simulink model "VFlexP_small"  (R2026a)
settings: Solver=ode23tb  StopTime=2  FixedStep=5e-5
model workspace (MAT data in the model file):
  DCop_DCBUCK : object (value not decoded)
  Grid_CCVSC_idx = [2; 3; 4; 5; 6; 7; 8; 9; 10; 11; 12]
  Grid_CCVSCs = 1
  Grid_CCVSCs_buses = 1
  Grid_CCVSCs_toM = [0 1 0 0 0 0 0 0 0 0 0 0 ... (781 elements, 71x11)]
  Grid_C_Lines = 0
  Grid_Cbuses = [0.00666666666667 0.00666666666667]
  Grid_DC : object (value not decoded)
  Grid_DCop_DCBUCK : object (value not decoded)
  Grid_DCop_DC_PES : object (value not decoded)
  Grid_DFIGs = 1
  Grid_DFIGs_buses = 1
  Grid_DGs : string (value not decoded)
  Grid_From_buses = 1
  Grid_GFls = 1
  Grid_GFls_buses = 1
  Grid_GFr_idx = 1
  Grid_GFrs = 1
  Grid_GFrs_buses = 1
  Grid_GFrs_toM = [1; 0]
  Grid_IG_idx = 1
  Grid_IGs = 1
  Grid_IGs_buses = 1
  Grid_IGs_toM = [1; 0; 0]
  Grid_L_Lines = 0.05
  Grid_L_Loads = [0 0]
  Grid_Lines_fromM : object (value not decoded)
  Grid_Lines_toM : object (value not decoded)
  Grid_Load_buses = [1; 2]
  Grid_Load_busesDC = []
  Grid_MSGs = 1
  Grid_MSGs_buses = 1
  Grid_Nbuses = 2
  Grid_PQ_gen = 3
  Grid_Ploads = [0.0075 0.0075]
  Grid_PloadsDC = []
  Grid_Ps_lf = 0.51232912
  Grid_Qloads = [0 0]
  Grid_Qs_lf = -0.00723209333333
  Grid_R_Lines = 0.005
  Grid_R_Loads = [2 2]
  Grid_R_Loads_DC = 0
  Grid_Rcf = [150 150]
  Grid_SCs = 1
  Grid_SCs_buses = 1
  Grid_SG_idx = 1
  Grid_SGs = 1
  Grid_SGs_buses = 1
  Grid_SGs_toM = [1; 0]
  Grid_To_buses = 2
  Grid_VCVSC_idx = [1; 2; 3; 4; 5; 6; 7; 8; 9; 10; 11; 12]
  Grid_VCVSCs = 1
  Grid_VCVSCs_buses = [1; 2; 3; 6; 8; 9; 12; 58; 59; 60; 63; 65]
  Grid_VCVSCs_toM = [1 0 0 0 0 0 0 0 0 0 0 0 ... (852 elements, 71x12)]
  Grid_VSM_idx = 2
  Grid_VSMs = 1
  Grid_VSMs_buses = 1
  Grid_VSMs_toM = [0; 1]
  Grid_admitt_matrix = [2.15353135314-19.7953135314i  -1.9801980198+19.801980198i; -1.9801980198+19.801980198i  2.15353135314-19.7953135314i]
  Grid_admitt_matrix_noloads = [1.98686468647-19.7953135314i  -1.9801980198+19.801980198i; -1.9801980198+19.801980198i  1.98686468647-19.7953135314i]
  Grid_bus = [1; 2]
  Grid_busDC_complexity = 1
  Grid_busDC_complexity_PF = 2
  Grid_bus_complexity = [1 1]
  Grid_bus_complexity_PF = [1 1]
  Grid_buses_lf = 1
  Grid_conductance_matrix = 0.00666666666667
  Grid_conductance_matrix_noloads = 0.00666666666667
  Grid_fref : object (value not decoded)
  Grid_gen_static_params : mBase (value not decoded)
  Grid_iPs_lf = 1.95187031336
  Grid_iQs_lf = -138.272551792
  Grid_iadmitt_matrix = [2.88165849328-0.0982918688642i  2.87905051706-0.123273862303i; 2.87905051706-0.123273862303i  2.88165849328-0.0982918688642i]
  Grid_iadmitt_matrix_noloads = [37.5012524798-37.4874983544i  37.4987475202-37.5125016456i; 37.4987475202-37.5125016456i  37.5012524798-37.4874983544i]
  Grid_iconductance_matrix = 150
  Grid_iconductance_matrix_noloads = 150
  Grid_init_OK_bool = 1
  Grid_intconv_PF : object (value not decoded)
  Grid_lf_op : op_report (value not decoded)
  Grid_lineDC_complexity = []
  Grid_lineDC_complexity_PF = []
  Grid_line_complexity = 1
  Grid_line_complexity_PF = 3
  Grid_loadDC_complexity = []
  Grid_loadDC_complexity_PF = []
  Grid_load_complexity = [3 3]
  Grid_load_complexity_PF = [4 4]
  Grid_opDC_CCVSC : object (value not decoded)
  Grid_opDC_VSM : object (value not decoded)
  Grid_opGFr : object (value not decoded)
  Grid_opVCVSC : object (value not decoded)
  Grid_op_CCVSC : object (value not decoded)
  Grid_op_IG : object (value not decoded)
  Grid_op_SG : object (value not decoded)
  Grid_op_VSM : object (value not decoded)
  Grid_shift_lines = 0
  Grid_tap_lines = 1
  Grid_v_buses_mod = [1 1]
  LinsysParamChangeStruct : Param1 (value not decoded)
  Lline = 0.01
  Rline = 1e-05
  linsys : object (value not decoded)
values from neighbouring files (symbols this model uses):
  block_idx = evalin(mdlWks, [bvarname Generators{i} '_idx'])    [fun_init_units_callback.m]
  Fb = areas    [fun_MATPOWER_to_Excel.m]
  Fi = evalin('base', get_param(block, 'Fi'))    [fun_init_GFr.m]    (also in fun_init_intconv_DC_VSM.m)
  Lf = evalin('base', get_param(block, 'Lf'))    [fun_init_GFr.m]    (also in fun_init_intconv_DC_VSM.m)
  Rf = evalin('base', get_param(block, 'Rf'))    [fun_init_GFr.m]    (also in fun_init_intconv_DC_VSM.m)
symbols that are objects in the model workspace (value not decoded): Grid_DCop_DC_PES, Grid_DCop_DCBUCK, Grid_op_CCVSC, Grid_op_IG, Grid_op_SG, Grid_op_VSM, Grid_opDC_CCVSC, Grid_opDC_VSM, Grid_opGFr, Grid_opVCVSC
undefined symbols (not defined in the file or in its folder): block_buses_DC, CCVSC_idx, Cf, costs, costs2, DFIGs_nodes, DiscIntNeverNeededParam, entity, From_nodes, grid_linsys, Grid_op_DFIG, Grid_op_DFIG_PQ, Grid_op_MSG, Grid_op_SC, Grid_op_VCVSC, Hv, initial_states_grid, Kic, Kiv, Kp_theta, Kp_w, Kpc, Kpv, last_send, Lc, m, Matrix_flux_to_i, mD, mp, MSGs_buses, Nbuses_DC, nq, op_VCVSC, Psche, Rc, rkq1, rkq2, SCs_buses, SCs_nodes, sec_control_structure, set_asked, set_DG_up, set_extra_satur, set_sending_cost, SGs_buses, SGs_nodes, Tf, To_nodes, VI_L, VI_R, WOF_Tf, xkq1, xkq2
libraries: simulink x1045, eeGeneralControl x12, eeTransforms x1, sl_discontinuities x1
(part 34 of 50)

== system VFlexP_small/Grid/Dynamic/Tertiary Control/MAS messages/ID6/Simulink Function14 ==
  set_cost_info : TriggerPort  TriggerType=function-call  IsSimulinkFunction=on  FunctionName=set_cost_info  FunctionVisibility=scoped  VariantControl=(inherit)
  cost : ArgIn  ArgumentName=cost
  Output : Outport
  wires:
  cost/1 -> Output/1

== system VFlexP_small/Grid/Dynamic/Tertiary Control/MAS messages/ID6/Simulink Function15 ==
  set_DG_up : TriggerPort  TriggerType=function-call  IsSimulinkFunction=on  FunctionName=set_DG_up  FunctionVisibility=scoped  VariantControl=(inherit)
  u : ArgIn  DisableCoverage=on  ArgumentName=u
  Output : Outport
  wires:
  u/1 -> Output/1

== system VFlexP_small/Grid/Dynamic/Tertiary Control/MAS messages/ID6/Simulink Function16 ==
  Input1 : Inport
  get_DG_up : TriggerPort  TriggerType=function-call  IsSimulinkFunction=on  FunctionName=get_DG_up  FunctionVisibility=scoped  VariantControl=(inherit)
  value : ArgOut  OutDataTypeStr=boolean  ArgumentName=value
  wires:
  Input1/1 -> value/1

== system VFlexP_small/Grid/Dynamic/Tertiary Control/MAS messages/ID6/Simulink Function17 ==
  set_neigh_ID : TriggerPort  TriggerType=function-call  IsSimulinkFunction=on  FunctionName=set_neigh_ID  FunctionVisibility=scoped  VariantControl=(inherit)
  u : ArgIn  DisableCoverage=on  ArgumentName=u
  Output : Outport
  wires:
  u/1 -> Output/1

== system VFlexP_small/Grid/Dynamic/Tertiary Control/MAS messages/ID6/Simulink Function18 ==
  Input1 : Inport
  get_neigh_ID : TriggerPort  TriggerType=function-call  IsSimulinkFunction=on  FunctionName=get_neigh_ID  FunctionVisibility=scoped  VariantControl=(inherit)
  value : ArgOut  ArgumentName=value
  wires:
  Input1/1 -> value/1

== system VFlexP_small/Grid/Dynamic/Tertiary Control/MAS messages/ID6/Simulink Function19 ==
  set_neigh_Opt : TriggerPort  TriggerType=function-call  IsSimulinkFunction=on  FunctionName=set_neigh_Opt  FunctionVisibility=scoped  VariantControl=(inherit)
  u : ArgIn  DisableCoverage=on  ArgumentName=u
  Output : Outport
  wires:
  u/1 -> Output/1

== system VFlexP_small/Grid/Dynamic/Tertiary Control/MAS messages/ID6/Simulink Function2 ==
  unpackage : TriggerPort  TriggerType=function-call  IsSimulinkFunction=on  FunctionName=unpackage  FunctionVisibility=scoped  VariantControl=(inherit)
  IC1 : InitialCondition
  IC2 : InitialCondition
  IC3 : InitialCondition  Value=v_buses_mod(buses_lf(IDnumber))
  IC4 : InitialCondition
  mpP~ : ArgIn  ArgumentName=P_s
  nqQ~ : ArgIn  Port=2  ArgumentName=Q_s
  v : ArgIn  Port=3  ArgumentName=v
  omega : ArgIn  Port=4  ArgumentName=omega
  Output2 : Outport
  Output3 : Outport  Port=2
  Output4 : Outport  Port=3
  Output5 : Outport  Port=4
  wires:
  omega/1 -> IC4/1  "omega"
  v/1 -> IC3/1  "v"
  nqQ~/1 -> IC2/1  "Q_s"
  mpP~/1 -> IC1/1  "P_s"
  IC1/1 -> Output2/1
  IC2/1 -> Output3/1
  IC4/1 -> Output5/1
  IC3/1 -> Output4/1

== system VFlexP_small/Grid/Dynamic/Tertiary Control/MAS messages/ID6/Simulink Function20 ==
  Input1 : Inport
  get_neigh_Opt : TriggerPort  TriggerType=function-call  IsSimulinkFunction=on  FunctionName=get_neigh_Opt  FunctionVisibility=scoped  VariantControl=(inherit)
  value : ArgOut  ArgumentName=value
  wires:
  Input1/1 -> value/1

== system VFlexP_small/Grid/Dynamic/Tertiary Control/MAS messages/ID6/Simulink Function21 ==
  set_sum_neigh_left : TriggerPort  TriggerType=function-call  IsSimulinkFunction=on  FunctionName=set_sum_neigh_left  FunctionVisibility=scoped  VariantControl=(inherit)
  u : ArgIn  DisableCoverage=on  ArgumentName=u
  Output : Outport
  wires:
  u/1 -> Output/1

== system VFlexP_small/Grid/Dynamic/Tertiary Control/MAS messages/ID6/Simulink Function22 ==
  set_Opt : TriggerPort  TriggerType=function-call  IsSimulinkFunction=on  FunctionName=set_Opt  FunctionVisibility=scoped  VariantControl=(inherit)
  u : ArgIn  DisableCoverage=on  ArgumentName=u
  Output : Outport
  wires:
  u/1 -> Output/1

== system VFlexP_small/Grid/Dynamic/Tertiary Control/MAS messages/ID6/Simulink Function23 ==
  Input1 : Inport
  get_sum_neigh_left : TriggerPort  TriggerType=function-call  IsSimulinkFunction=on  FunctionName=get_sum_neigh_left  FunctionVisibility=scoped  VariantControl=(inherit)
  value : ArgOut  ArgumentName=value
  wires:
  Input1/1 -> value/1  "sum_neigh_left"

== system VFlexP_small/Grid/Dynamic/Tertiary Control/MAS messages/ID6/Simulink Function24 ==
  set_decision_turn : TriggerPort  TriggerType=function-call  IsSimulinkFunction=on  FunctionName=set_decision_turn  FunctionVisibility=scoped  VariantControl=(inherit)
  u : ArgIn  DisableCoverage=on  ArgumentName=u
  Output : Outport
  wires:
  u/1 -> Output/1

== system VFlexP_small/Grid/Dynamic/Tertiary Control/MAS messages/ID6/Simulink Function25 ==
  Input1 : Inport
  get_ID : TriggerPort  TriggerType=function-call  IsSimulinkFunction=on  FunctionName=get_ID  FunctionVisibility=scoped  VariantControl=(inherit)
  value : ArgOut  ArgumentName=value
  wires:
  Input1/1 -> value/1

== system VFlexP_small/Grid/Dynamic/Tertiary Control/MAS messages/ID6/Simulink Function26 ==
  set_Neighbor_ID : TriggerPort  TriggerType=function-call  IsSimulinkFunction=on  FunctionName=set_Neighbor_ID  FunctionVisibility=scoped  VariantControl=(inherit)
  u : ArgIn  DisableCoverage=on  ArgumentName=u
  Output : Outport
  wires:
  u/1 -> Output/1

== system VFlexP_small/Grid/Dynamic/Tertiary Control/MAS messages/ID6/Simulink Function27 ==
  set_original_Opt : TriggerPort  TriggerType=function-call  IsSimulinkFunction=on  FunctionName=set_original_Opt  FunctionVisibility=scoped  VariantControl=(inherit)
  u : ArgIn  DisableCoverage=on  ArgumentName=u
  Output : Outport
  wires:
  u/1 -> Output/1

== system VFlexP_small/Grid/Dynamic/Tertiary Control/MAS messages/ID6/Simulink Function28 ==
  set_Neighbor_Opt : TriggerPort  TriggerType=function-call  IsSimulinkFunction=on  FunctionName=set_Neighbor_Opt  FunctionVisibility=scoped  VariantControl=(inherit)
  u : ArgIn  DisableCoverage=on  ArgumentName=u
  Output : Outport
  wires:
  u/1 -> Output/1

== system VFlexP_small/Grid/Dynamic/Tertiary Control/MAS messages/ID6/Simulink Function29 ==
  Input1 : Inport
  get_original_Opt : TriggerPort  TriggerType=function-call  IsSimulinkFunction=on  FunctionName=get_original_Opt  FunctionVisibility=scoped  VariantControl=(inherit)
  value : ArgOut  ArgumentName=value
  wires:
  Input1/1 -> value/1

== system VFlexP_small/Grid/Dynamic/Tertiary Control/MAS messages/ID6/Simulink Function3 ==
  Input1 : Inport
  get_following : TriggerPort  TriggerType=function-call  IsSimulinkFunction=on  FunctionName=get_following  FunctionVisibility=scoped  VariantControl=(inherit)
  value : ArgOut  ArgumentName=value
  wires:
  Input1/1 -> value/1

== system VFlexP_small/Grid/Dynamic/Tertiary Control/MAS messages/ID6/Simulink Function30 ==
  set_original_ID : TriggerPort  TriggerType=function-call  IsSimulinkFunction=on  FunctionName=set_original_ID  FunctionVisibility=scoped  VariantControl=(inherit)
  u : ArgIn  DisableCoverage=on  ArgumentName=u
  Output : Outport
  wires:
  u/1 -> Output/1

== system VFlexP_small/Grid/Dynamic/Tertiary Control/MAS messages/ID6/Simulink Function31 ==
  Input1 : Inport
  get_original_ID : TriggerPort  TriggerType=function-call  IsSimulinkFunction=on  FunctionName=get_original_ID  FunctionVisibility=scoped  VariantControl=(inherit)
  value : ArgOut  ArgumentName=value
  wires:
  Input1/1 -> value/1

== system VFlexP_small/Grid/Dynamic/Tertiary Control/MAS messages/ID6/Simulink Function32 ==
  set_asked : TriggerPort  TriggerType=function-call  IsSimulinkFunction=on  FunctionName=set_asked  FunctionVisibility=scoped  VariantControl=(inherit)
  u : ArgIn  DisableCoverage=on  ArgumentName=u
  Output : Outport
  wires:
  u/1 -> Output/1

== system VFlexP_small/Grid/Dynamic/Tertiary Control/MAS messages/ID6/Simulink Function33 ==
  Input : Inport
  get_cost_P : TriggerPort  TriggerType=function-call  IsSimulinkFunction=on  FunctionName=get_cost_P  FunctionVisibility=scoped  VariantControl=(inherit)
  y : ArgOut  DisableCoverage=on  ArgumentName=y
  wires:
  Input/1 -> y/1

== system VFlexP_small/Grid/Dynamic/Tertiary Control/MAS messages/ID6/Simulink Function34 ==
  Input1 : Inport
  get_asked : TriggerPort  TriggerType=function-call  IsSimulinkFunction=on  FunctionName=get_asked  FunctionVisibility=scoped  VariantControl=(inherit)
  value : ArgOut  ArgumentName=value
  wires:
  Input1/1 -> value/1

== system VFlexP_small/Grid/Dynamic/Tertiary Control/MAS messages/ID6/Simulink Function35 ==
  Input : Inport
  get_extra_satur : TriggerPort  TriggerType=function-call  IsSimulinkFunction=on  FunctionName=get_extra_satur  FunctionVisibility=scoped  VariantControl=(inherit)
  y : ArgOut  ArgumentName=y
  wires:
  Input/1 -> y/1

== system VFlexP_small/Grid/Dynamic/Tertiary Control/MAS messages/ID6/Simulink Function36 ==
  Input1 : Inport
  get_Opt : TriggerPort  TriggerType=function-call  IsSimulinkFunction=on  FunctionName=get_Opt  FunctionVisibility=scoped  VariantControl=(inherit)
  value : ArgOut  ArgumentName=value
  wires:
  Input1/1 -> value/1

== system VFlexP_small/Grid/Dynamic/Tertiary Control/MAS messages/ID6/Simulink Function37 ==
  set_sending_cost : TriggerPort  TriggerType=function-call  IsSimulinkFunction=on  FunctionName=set_sending_cost  FunctionVisibility=scoped  VariantControl=(inherit)
  u : ArgIn  DisableCoverage=on  ArgumentName=u
  Output : Outport
  wires:
  u/1 -> Output/1

== system VFlexP_small/Grid/Dynamic/Tertiary Control/MAS messages/ID6/Simulink Function38 ==
  set_extra_satur : TriggerPort  TriggerType=function-call  IsSimulinkFunction=on  FunctionName=set_extra_satur  FunctionVisibility=scoped  VariantControl=(inherit)
  u : ArgIn  DisableCoverage=on  ArgumentName=u
  Output : Outport
  wires:
  u/1 -> Output/1

== system VFlexP_small/Grid/Dynamic/Tertiary Control/MAS messages/ID6/Simulink Function4 ==
  Input2 : Inport
  last_send : TriggerPort  TriggerType=function-call  IsSimulinkFunction=on  FunctionName=last_send  FunctionVisibility=scoped  VariantControl=(inherit)
  u : ArgIn  DisableCoverage=on  ArgumentName=v
  u1 : ArgIn  DisableCoverage=on  Port=2  ArgumentName=omega
  Output : Outport
  Output1 : Outport  Port=2
  time : Outport  Port=3
  wires:
  Input2/1 -> time/1  "time"
  u1/1 -> Output1/1  "omega"
  u/1 -> Output/1  "v"

== system VFlexP_small/Grid/Dynamic/Tertiary Control/MAS messages/ID6/Simulink Function5 ==
  send_to : TriggerPort  TriggerType=function-call  IsSimulinkFunction=on  FunctionName=send_to  FunctionVisibility=scoped  VariantControl=(inherit)
  u : ArgIn  DisableCoverage=on  ArgumentName=u
  Output : Outport
  wires:
  u/1 -> Output/1

== system VFlexP_small/Grid/Dynamic/Tertiary Control/MAS messages/ID6/Simulink Function6 ==
  Input1 : Inport
  Dest : TriggerPort  TriggerType=function-call  IsSimulinkFunction=on  FunctionName=Dest  FunctionVisibility=scoped  VariantControl=(inherit)
  Dest~ : ArgOut  DisableCoverage=on  ArgumentName=Dest
  wires:
  Input1/1 -> Dest~/1  "Dest"

== system VFlexP_small/Grid/Dynamic/Tertiary Control/MAS messages/ID6/Simulink Function7 ==
  set_following : TriggerPort  TriggerType=function-call  IsSimulinkFunction=on  FunctionName=set_following  FunctionVisibility=scoped  VariantControl=(inherit)
  u : ArgIn  DisableCoverage=on  ArgumentName=u
  Output : Outport
  wires:
  u/1 -> Output/1

== system VFlexP_small/Grid/Dynamic/Tertiary Control/MAS messages/ID6/Simulink Function8 ==
  type : TriggerPort  TriggerType=function-call  IsSimulinkFunction=on  FunctionName=type  FunctionVisibility=scoped  VariantControl=(inherit)
  Compare To Constant : simulink/Logic and Bit Operations/Compare To Constant  relop=~=  const=0  OutDataTypeStr=boolean  ZeroCross=off
  Send : Send  OutputPortMessageModes=m  ShowEnablePort=on
      settings: InputPortMap=e0,u1
  u : ArgIn  DisableCoverage=on  ArgumentName=u
  type_out : Outport
  trigger : Outport  Port=2
  wires:
  Send/1 -> trigger/1
  Compare To Constant/1 -> Send/2, Send/1
  u/1 -> type_out/1, Compare To Constant/1

== system VFlexP_small/Grid/Dynamic/Tertiary Control/MAS messages/ID6/Simulink Function9 ==
  Input1 : Inport
  get_leader : TriggerPort  TriggerType=function-call  IsSimulinkFunction=on  FunctionName=get_leader  FunctionVisibility=scoped  VariantControl=(inherit)
  value : ArgOut  ArgumentName=value
  wires:
  Input1/1 -> value/1

== system VFlexP_small/Grid/Dynamic/Tertiary Control/MAS messages/ID6/Subsystem ==
  In1 : Inport
  In3 : Inport  Port=2
  In4 : Inport  Port=3
  AND11 : Logic  IconShape=distinctive  AllPortsSameDT=off  OutDataTypeStr=boolean
  AND9 : Logic  IconShape=distinctive  AllPortsSameDT=off  OutDataTypeStr=boolean
  Compare To Zero : simulink/Logic and Bit Operations/Compare To Zero  relop=>  OutDataTypeStr=boolean
  Compare To Zero1 : simulink/Logic and Bit Operations/Compare To Zero  relop=<  OutDataTypeStr=boolean
  NOT : Logic  Operator=NOT  IconShape=distinctive  AllPortsSameDT=off  OutDataTypeStr=boolean
  OR4 : Logic  Operator=OR  IconShape=distinctive  AllPortsSameDT=off  OutDataTypeStr=boolean
  Relational Operator2 : RelationalOperator  Operator=<  OutDataTypeStr=boolean  RndMeth=Simplest  InputSameDT=off
  Relational Operator3 : RelationalOperator  Operator=>  OutDataTypeStr=boolean  RndMeth=Simplest  InputSameDT=off
  Out1 : Outport
  inf_satur : Outport  Port=2
  wires:
  In1/1 -> Compare To Zero/1, Compare To Zero1/1
  OR4/1 -> NOT/1
  Relational Operator2/1 -> AND9/1
  AND9/1 -> OR4/1
  In4/1 -> Relational Operator2/1, Relational Operator3/1
  AND11/1 -> inf_satur/1, OR4/2
  Relational Operator3/1 -> AND11/1
  In3/1 -> Relational Operator2/2, Relational Operator3/2
  Compare To Zero1/1 -> AND11/2
  Compare To Zero/1 -> AND9/2
  NOT/1 -> Out1/1

== system VFlexP_small/Grid/Dynamic/Tertiary Control/MAS messages/ID6/Triggered Subsystem ==
  In1 : Inport
  Trigger : TriggerPort  VariantControl=(inherit)
  Out1 : Outport
  wires:
  In1/1 -> Out1/1

== system VFlexP_small/Grid/Dynamic/Tertiary Control/MAS messages/ID6/Triggered Subsystem1 ==
  In1 : Inport
  Trigger : TriggerPort  VariantControl=(inherit)
  Out1 : Outport
  wires:
  In1/1 -> Out1/1

== system VFlexP_small/Grid/Dynamic/Tertiary Control/MAS messages/ID6/Triggered Subsystem2 ==
  In1 : Inport
  Trigger : TriggerPort  VariantControl=(inherit)
  Out1 : Outport
  wires:
  In1/1 -> Out1/1

== system VFlexP_small/Grid/Dynamic/Tertiary Control/MAS messages/ID6/Triggered Subsystem3 ==
  Trigger : TriggerPort  VariantControl=(inherit)
  One : Constant  OutDataTypeStr=Inherit: Inherit via back propagation
  Send7 : Send  OutputPortMessageModes=m  ShowEnablePort=on
      settings: InputPortMap=e0,u1
  Out1 : Outport
  wires:
  Send7/1 -> Out1/1
  One/1 -> Send7/2, Send7/1

== system VFlexP_small/Grid/Dynamic/Tertiary Control/MAS messages/ID6/Triggered Subsystem4 ==
  In1 : Inport
  Trigger : TriggerPort  VariantControl=(inherit)
  Out1 : Outport
  wires:
  In1/1 -> Out1/1

== system VFlexP_small/Grid/Dynamic/Tertiary Control/MAS messages/ID6/Triggered Subsystem5 ==
  In1 : Inport
  Trigger : TriggerPort  TriggerType=falling  VariantControl=(inherit)
  Constant : Constant
  IC : InitialCondition  Value=0
  Out1 : Outport
  Output : Outport  Port=2
  wires:
  In1/1 -> Out1/1
  Constant/1 -> IC/1
  IC/1 -> Output/1

== system VFlexP_small/Grid/Dynamic/Tertiary Control/MAS messages/ID6/Triggered Subsystem6 ==
  In1 : Inport
  Trigger : TriggerPort  VariantControl=(inherit)
  Out1 : Outport
  wires:
  In1/1 -> Out1/1

== system VFlexP_small/Grid/Dynamic/Tertiary Control/MAS messages/ID6/ramp ==
  connected : Inport
  time : Inport  Port=2
  Clock5 : Clock
      settings: DisableCoverage=on
  Gain : Gain  Gain=0.05
  Product : Product
  Sum6 : Sum  DisableCoverage=on  Inputs=|+-  InputSameDT=on  SaturateOnIntegerOverflow=on  OutDataTypeStr=Inherit: Same as first input
  Out1 : Outport
  wires:
  connected/1 -> Product/1
  Product/1 -> Gain/1
  Gain/1 -> Out1/1
  Sum6/1 -> Product/2
  time/1 -> Sum6/2
  Clock5/1 -> Sum6/1

== system VFlexP_small/Grid/Dynamic/Tertiary Control/MAS messages/ID6/time ==
  time : Inport
  Trigger : TriggerPort  VariantControl=(inherit)
  Out1 : Outport
  wires:
  time/1 -> Out1/1

== system VFlexP_small/Grid/Dynamic/Tertiary Control/MAS messages/ID7/Compare to last ==
  Output : Inport
  In4 : Inport  Port=2
  In1 : Inport  Port=3
  Output1 : Inport  Port=4
  time_last : Inport  Port=5
  com : Inport  Port=6
  AND : Logic  Inputs=3  IconShape=distinctive  AllPortsSameDT=off  OutDataTypeStr=boolean
  Abs : Abs  ZeroCross=off  SaturateOnIntegerOverflow=off
  Abs1 : Abs  ZeroCross=off  SaturateOnIntegerOverflow=off
  Clock1 : Clock
  Compare To Constant1 : simulink/Logic and Bit Operations/Compare To Constant  relop=>  const=1  OutDataTypeStr=boolean  ZeroCross=off
  Compare To Constant2 : simulink/Logic and Bit Operations/Compare To Constant  relop=>  const=1e-2  OutDataTypeStr=boolean  ZeroCross=off
  Gain : Gain  Gain=1e4
  Gain1 : Gain  Gain=1e5
  Send1 : Send  OutputPortMessageModes=m  ShowEnablePort=on
      settings: InputPortMap=e0,u1
  Sum : Sum  Inputs=|+-
  Sum1 : Sum  Inputs=|+-
  Sum2 : Sum  Inputs=|++
  Sum5 : Sum  Inputs=|+-
  Trigger : Outport
  wires:
  com/1 -> AND/3
  Gain1/1 -> Sum2/2
  Gain/1 -> Sum2/1
  Compare To Constant1/1 -> AND/1
  Sum2/1 -> Compare To Constant1/1
  Abs1/1 -> Gain1/1
  Compare To Constant2/1 -> AND/2
  Clock1/1 -> Sum1/1  "time"
  time_last/1 -> Sum1/2  "time_last"
  Sum1/1 -> Compare To Constant2/1
  AND/1 -> Send1/2, Send1/1
  In4/1 -> Sum5/2  "last_omega"
  Sum5/1 -> Abs1/1
  Abs/1 -> Gain/1
  Sum/1 -> Abs/1
  Send1/1 -> Trigger/1
  Output1/1 -> Sum5/1  "omega"
  In1/1 -> Sum/1  "v"
  Output/1 -> Sum/2  "last_v"

== system VFlexP_small/Grid/Dynamic/Tertiary Control/MAS messages/ID7/Send to neighbor ==
  note: 1) Add Subsystem or Model blocks as valid variant choices.
      | 2) You cannot connect blocks at this level. At simulation, connectivity is automatically
      | determined, based on the active variant and port name matching.
  Message : Inport
  five : Subsystem  VariantControl=five
  four : Subsystem  VariantControl=four
  one : Subsystem  VariantControl=one
  three : Subsystem  VariantControl=three
  two : Subsystem  VariantControl=two

== system VFlexP_small/Grid/Dynamic/Tertiary Control/MAS messages/ID7/Send to neighbor1 ==
  note: 1) Add Subsystem or Model blocks as valid variant choices.
      | 2) You cannot connect blocks at this level. At simulation, connectivity is automatically
      | determined, based on the active variant and port name matching.
  Message : Inport
  five : Subsystem  VariantControl=five
  four : Subsystem  VariantControl=four
  one : Subsystem  VariantControl=one
  three : Subsystem  VariantControl=three
  two : Subsystem  VariantControl=two

== system VFlexP_small/Grid/Dynamic/Tertiary Control/MAS messages/ID7/Send to neighbor2 ==
  note: 1) Add Subsystem or Model blocks as valid variant choices.
      | 2) You cannot connect blocks at this level. At simulation, connectivity is automatically
      | determined, based on the active variant and port name matching.
  Message : Inport
  five : Subsystem  VariantControl=five
  four : Subsystem  VariantControl=four
  one : Subsystem  VariantControl=one
  three : Subsystem  VariantControl=three
  two : Subsystem  VariantControl=two

== system VFlexP_small/Grid/Dynamic/Tertiary Control/MAS messages/ID7/Simulink Function ==
  Input : Inport
  get_cost : TriggerPort  TriggerType=function-call  IsSimulinkFunction=on  FunctionName=get_cost  FunctionVisibility=scoped  VariantControl=(inherit)
  y : ArgOut  DisableCoverage=on  ArgumentName=y
  wires:
  Input/1 -> y/1

== system VFlexP_small/Grid/Dynamic/Tertiary Control/MAS messages/ID7/Simulink Function1 ==
  Input1 : Inport
  Input2 : Inport  Port=2
  Input3 : Inport  Port=3
  Input4 : Inport  Port=4
  Input6 : Inport  Port=5
  Input5 : Inport  Port=6
  Input7 : Inport  Port=7
  Output : Inport  Port=8
  In9 : Inport  Port=9
  In10 : Inport  Port=10
  package : TriggerPort  TriggerType=function-call  IsSimulinkFunction=on  FunctionName=package  FunctionVisibility=scoped  VariantControl=(inherit)
  Source : ArgOut  DisableCoverage=on  ArgumentName=Source
  Dest : ArgOut  DisableCoverage=on  Port=2  ArgumentName=Dest
  P_s : ArgOut  DisableCoverage=on  Port=3  ArgumentName=P_s
  nqQ : ArgOut  DisableCoverage=on  Port=4  ArgumentName=Q_s
  v : ArgOut  DisableCoverage=on  Port=5  ArgumentName=v
  omega : ArgOut  DisableCoverage=on  Port=6  ArgumentName=omega
  type : ArgOut  DisableCoverage=on  Port=7  ArgumentName=type
  Opt : ArgOut  Port=8  ArgumentName=Opt
  Neighbor_ID : ArgOut  Port=9  ArgumentName=Neighbor_ID
  Neighbor_Opt : ArgOut  Port=10  ArgumentName=Neighbor_Opt
  wires:
  In9/1 -> Neighbor_ID/1  "Neighbor_ID"
  In10/1 -> Neighbor_Opt/1  "Neighbor_Opt"
  Output/1 -> Opt/1  "Opt"
  Input7/1 -> type/1  "type"
  Input5/1 -> omega/1  "omega"
  Input6/1 -> v/1  "v"
  Input4/1 -> nqQ/1  "Q_s"
  Input3/1 -> P_s/1  "P_s"
  Input2/1 -> Dest/1  "Dest"
  Input1/1 -> Source/1  "Source"

== system VFlexP_small/Grid/Dynamic/Tertiary Control/MAS messages/ID7/Simulink Function10 ==
  set_leader : TriggerPort  TriggerType=function-call  IsSimulinkFunction=on  FunctionName=set_leader  FunctionVisibility=scoped  VariantControl=(inherit)
  u : ArgIn  DisableCoverage=on  ArgumentName=u
  Output : Outport
  wires:
  u/1 -> Output/1

== system VFlexP_small/Grid/Dynamic/Tertiary Control/MAS messages/ID7/Simulink Function11 ==
  Input1 : Inport
  get_sending : TriggerPort  TriggerType=function-call  IsSimulinkFunction=on  FunctionName=get_sending  FunctionVisibility=scoped  VariantControl=(inherit)
  value : ArgOut  ArgumentName=value
  wires:
  Input1/1 -> value/1

== system VFlexP_small/Grid/Dynamic/Tertiary Control/MAS messages/ID7/Simulink Function12 ==
  set_sending : TriggerPort  TriggerType=function-call  IsSimulinkFunction=on  FunctionName=set_sending  FunctionVisibility=scoped  VariantControl=(inherit)
  u : ArgIn  DisableCoverage=on  ArgumentName=u
  Output : Outport
  wires:
  u/1 -> Output/1

== system VFlexP_small/Grid/Dynamic/Tertiary Control/MAS messages/ID7/Simulink Function13 ==
  Input1 : Inport
  get_type : TriggerPort  TriggerType=function-call  IsSimulinkFunction=on  FunctionName=get_type  FunctionVisibility=scoped  VariantControl=(inherit)
  value : ArgOut  ArgumentName=type
  wires:
  Input1/1 -> value/1  "type"

== system VFlexP_small/Grid/Dynamic/Tertiary Control/MAS messages/ID7/Simulink Function14 ==
  set_cost_info : TriggerPort  TriggerType=function-call  IsSimulinkFunction=on  FunctionName=set_cost_info  FunctionVisibility=scoped  VariantControl=(inherit)
  cost : ArgIn  ArgumentName=cost
  Output : Outport
  wires:
  cost/1 -> Output/1

== system VFlexP_small/Grid/Dynamic/Tertiary Control/MAS messages/ID7/Simulink Function15 ==
  set_DG_up : TriggerPort  TriggerType=function-call  IsSimulinkFunction=on  FunctionName=set_DG_up  FunctionVisibility=scoped  VariantControl=(inherit)
  u : ArgIn  DisableCoverage=on  ArgumentName=u
  Output : Outport
  wires:
  u/1 -> Output/1

== system VFlexP_small/Grid/Dynamic/Tertiary Control/MAS messages/ID7/Simulink Function16 ==
  Input1 : Inport
  get_DG_up : TriggerPort  TriggerType=function-call  IsSimulinkFunction=on  FunctionName=get_DG_up  FunctionVisibility=scoped  VariantControl=(inherit)
  value : ArgOut  OutDataTypeStr=boolean  ArgumentName=value
  wires:
  Input1/1 -> value/1

== system VFlexP_small/Grid/Dynamic/Tertiary Control/MAS messages/ID7/Simulink Function17 ==
  set_neigh_ID : TriggerPort  TriggerType=function-call  IsSimulinkFunction=on  FunctionName=set_neigh_ID  FunctionVisibility=scoped  VariantControl=(inherit)
  u : ArgIn  DisableCoverage=on  ArgumentName=u
  Output : Outport
  wires:
  u/1 -> Output/1

== system VFlexP_small/Grid/Dynamic/Tertiary Control/MAS messages/ID7/Simulink Function18 ==
  Input1 : Inport
  get_neigh_ID : TriggerPort  TriggerType=function-call  IsSimulinkFunction=on  FunctionName=get_neigh_ID  FunctionVisibility=scoped  VariantControl=(inherit)
  value : ArgOut  ArgumentName=value
  wires:
  Input1/1 -> value/1

== system VFlexP_small/Grid/Dynamic/Tertiary Control/MAS messages/ID7/Simulink Function19 ==
  set_neigh_Opt : TriggerPort  TriggerType=function-call  IsSimulinkFunction=on  FunctionName=set_neigh_Opt  FunctionVisibility=scoped  VariantControl=(inherit)
  u : ArgIn  DisableCoverage=on  ArgumentName=u
  Output : Outport
  wires:
  u/1 -> Output/1

== system VFlexP_small/Grid/Dynamic/Tertiary Control/MAS messages/ID7/Simulink Function2 ==
  unpackage : TriggerPort  TriggerType=function-call  IsSimulinkFunction=on  FunctionName=unpackage  FunctionVisibility=scoped  VariantControl=(inherit)
  IC1 : InitialCondition
  IC2 : InitialCondition
  IC3 : InitialCondition  Value=v_buses_mod(buses_lf(IDnumber))
  IC4 : InitialCondition
  mpP~ : ArgIn  ArgumentName=P_s
  nqQ~ : ArgIn  Port=2  ArgumentName=Q_s
  v : ArgIn  Port=3  ArgumentName=v
  omega : ArgIn  Port=4  ArgumentName=omega
  Output2 : Outport
  Output3 : Outport  Port=2
  Output4 : Outport  Port=3
  Output5 : Outport  Port=4
  wires:
  omega/1 -> IC4/1  "omega"
  v/1 -> IC3/1  "v"
  nqQ~/1 -> IC2/1  "Q_s"
  mpP~/1 -> IC1/1  "P_s"
  IC1/1 -> Output2/1
  IC2/1 -> Output3/1
  IC4/1 -> Output5/1
  IC3/1 -> Output4/1

== system VFlexP_small/Grid/Dynamic/Tertiary Control/MAS messages/ID7/Simulink Function20 ==
  Input1 : Inport
  get_neigh_Opt : TriggerPort  TriggerType=function-call  IsSimulinkFunction=on  FunctionName=get_neigh_Opt  FunctionVisibility=scoped  VariantControl=(inherit)
  value : ArgOut  ArgumentName=value
  wires:
  Input1/1 -> value/1

== system VFlexP_small/Grid/Dynamic/Tertiary Control/MAS messages/ID7/Simulink Function21 ==
  set_sum_neigh_left : TriggerPort  TriggerType=function-call  IsSimulinkFunction=on  FunctionName=set_sum_neigh_left  FunctionVisibility=scoped  VariantControl=(inherit)
  u : ArgIn  DisableCoverage=on  ArgumentName=u
  Output : Outport
  wires:
  u/1 -> Output/1

== system VFlexP_small/Grid/Dynamic/Tertiary Control/MAS messages/ID7/Simulink Function22 ==
  set_Opt : TriggerPort  TriggerType=function-call  IsSimulinkFunction=on  FunctionName=set_Opt  FunctionVisibility=scoped  VariantControl=(inherit)
  u : ArgIn  DisableCoverage=on  ArgumentName=u
  Output : Outport
  wires:
  u/1 -> Output/1

== system VFlexP_small/Grid/Dynamic/Tertiary Control/MAS messages/ID7/Simulink Function23 ==
  Input1 : Inport
  get_sum_neigh_left : TriggerPort  TriggerType=function-call  IsSimulinkFunction=on  FunctionName=get_sum_neigh_left  FunctionVisibility=scoped  VariantControl=(inherit)
  value : ArgOut  ArgumentName=value
  wires:
  Input1/1 -> value/1  "sum_neigh_left"

== system VFlexP_small/Grid/Dynamic/Tertiary Control/MAS messages/ID7/Simulink Function24 ==
  set_decision_turn : TriggerPort  TriggerType=function-call  IsSimulinkFunction=on  FunctionName=set_decision_turn  FunctionVisibility=scoped  VariantControl=(inherit)
  u : ArgIn  DisableCoverage=on  ArgumentName=u
  Output : Outport
  wires:
  u/1 -> Output/1

== system VFlexP_small/Grid/Dynamic/Tertiary Control/MAS messages/ID7/Simulink Function25 ==
  Input1 : Inport
  get_ID : TriggerPort  TriggerType=function-call  IsSimulinkFunction=on  FunctionName=get_ID  FunctionVisibility=scoped  VariantControl=(inherit)
  value : ArgOut  ArgumentName=value
  wires:
  Input1/1 -> value/1

== system VFlexP_small/Grid/Dynamic/Tertiary Control/MAS messages/ID7/Simulink Function26 ==
  set_Neighbor_ID : TriggerPort  TriggerType=function-call  IsSimulinkFunction=on  FunctionName=set_Neighbor_ID  FunctionVisibility=scoped  VariantControl=(inherit)
  u : ArgIn  DisableCoverage=on  ArgumentName=u
  Output : Outport
  wires:
  u/1 -> Output/1

== system VFlexP_small/Grid/Dynamic/Tertiary Control/MAS messages/ID7/Simulink Function27 ==
  set_original_Opt : TriggerPort  TriggerType=function-call  IsSimulinkFunction=on  FunctionName=set_original_Opt  FunctionVisibility=scoped  VariantControl=(inherit)
  u : ArgIn  DisableCoverage=on  ArgumentName=u
  Output : Outport
  wires:
  u/1 -> Output/1

== system VFlexP_small/Grid/Dynamic/Tertiary Control/MAS messages/ID7/Simulink Function28 ==
  set_Neighbor_Opt : TriggerPort  TriggerType=function-call  IsSimulinkFunction=on  FunctionName=set_Neighbor_Opt  FunctionVisibility=scoped  VariantControl=(inherit)
  u : ArgIn  DisableCoverage=on  ArgumentName=u
  Output : Outport
  wires:
  u/1 -> Output/1

== system VFlexP_small/Grid/Dynamic/Tertiary Control/MAS messages/ID7/Simulink Function29 ==
  Input1 : Inport
  get_original_Opt : TriggerPort  TriggerType=function-call  IsSimulinkFunction=on  FunctionName=get_original_Opt  FunctionVisibility=scoped  VariantControl=(inherit)
  value : ArgOut  ArgumentName=value
  wires:
  Input1/1 -> value/1

== system VFlexP_small/Grid/Dynamic/Tertiary Control/MAS messages/ID7/Simulink Function3 ==
  Input1 : Inport
  get_following : TriggerPort  TriggerType=function-call  IsSimulinkFunction=on  FunctionName=get_following  FunctionVisibility=scoped  VariantControl=(inherit)
  value : ArgOut  ArgumentName=value
  wires:
  Input1/1 -> value/1

== system VFlexP_small/Grid/Dynamic/Tertiary Control/MAS messages/ID7/Simulink Function30 ==
  set_original_ID : TriggerPort  TriggerType=function-call  IsSimulinkFunction=on  FunctionName=set_original_ID  FunctionVisibility=scoped  VariantControl=(inherit)
  u : ArgIn  DisableCoverage=on  ArgumentName=u
  Output : Outport
  wires:
  u/1 -> Output/1

== system VFlexP_small/Grid/Dynamic/Tertiary Control/MAS messages/ID7/Simulink Function31 ==
  Input1 : Inport
  get_original_ID : TriggerPort  TriggerType=function-call  IsSimulinkFunction=on  FunctionName=get_original_ID  FunctionVisibility=scoped  VariantControl=(inherit)
  value : ArgOut  ArgumentName=value
  wires:
  Input1/1 -> value/1

== system VFlexP_small/Grid/Dynamic/Tertiary Control/MAS messages/ID7/Simulink Function32 ==
  set_asked : TriggerPort  TriggerType=function-call  IsSimulinkFunction=on  FunctionName=set_asked  FunctionVisibility=scoped  VariantControl=(inherit)
  u : ArgIn  DisableCoverage=on  ArgumentName=u
  Output : Outport
  wires:
  u/1 -> Output/1

== system VFlexP_small/Grid/Dynamic/Tertiary Control/MAS messages/ID7/Simulink Function33 ==
  Input : Inport
  get_cost_P : TriggerPort  TriggerType=function-call  IsSimulinkFunction=on  FunctionName=get_cost_P  FunctionVisibility=scoped  VariantControl=(inherit)
  y : ArgOut  DisableCoverage=on  ArgumentName=y
  wires:
  Input/1 -> y/1

== system VFlexP_small/Grid/Dynamic/Tertiary Control/MAS messages/ID7/Simulink Function34 ==
  Input1 : Inport
  get_asked : TriggerPort  TriggerType=function-call  IsSimulinkFunction=on  FunctionName=get_asked  FunctionVisibility=scoped  VariantControl=(inherit)
  value : ArgOut  ArgumentName=value
  wires:
  Input1/1 -> value/1

== system VFlexP_small/Grid/Dynamic/Tertiary Control/MAS messages/ID7/Simulink Function35 ==
  Input : Inport
  get_extra_satur : TriggerPort  TriggerType=function-call  IsSimulinkFunction=on  FunctionName=get_extra_satur  FunctionVisibility=scoped  VariantControl=(inherit)
  y : ArgOut  ArgumentName=y
  wires:
  Input/1 -> y/1

== system VFlexP_small/Grid/Dynamic/Tertiary Control/MAS messages/ID7/Simulink Function36 ==
  Input1 : Inport
  get_Opt : TriggerPort  TriggerType=function-call  IsSimulinkFunction=on  FunctionName=get_Opt  FunctionVisibility=scoped  VariantControl=(inherit)
  value : ArgOut  ArgumentName=value
  wires:
  Input1/1 -> value/1

== system VFlexP_small/Grid/Dynamic/Tertiary Control/MAS messages/ID7/Simulink Function37 ==
  set_sending_cost : TriggerPort  TriggerType=function-call  IsSimulinkFunction=on  FunctionName=set_sending_cost  FunctionVisibility=scoped  VariantControl=(inherit)
  u : ArgIn  DisableCoverage=on  ArgumentName=u
  Output : Outport
  wires:
  u/1 -> Output/1

== system VFlexP_small/Grid/Dynamic/Tertiary Control/MAS messages/ID7/Simulink Function38 ==
  set_extra_satur : TriggerPort  TriggerType=function-call  IsSimulinkFunction=on  FunctionName=set_extra_satur  FunctionVisibility=scoped  VariantControl=(inherit)
  u : ArgIn  DisableCoverage=on  ArgumentName=u
  Output : Outport
  wires:
  u/1 -> Output/1

== system VFlexP_small/Grid/Dynamic/Tertiary Control/MAS messages/ID7/Simulink Function4 ==
  Input2 : Inport
  last_send : TriggerPort  TriggerType=function-call  IsSimulinkFunction=on  FunctionName=last_send  FunctionVisibility=scoped  VariantControl=(inherit)
  u : ArgIn  DisableCoverage=on  ArgumentName=v
  u1 : ArgIn  DisableCoverage=on  Port=2  ArgumentName=omega
  Output : Outport
  Output1 : Outport  Port=2
  time : Outport  Port=3
  wires:
  Input2/1 -> time/1  "time"
  u1/1 -> Output1/1  "omega"
  u/1 -> Output/1  "v"

== system VFlexP_small/Grid/Dynamic/Tertiary Control/MAS messages/ID7/Simulink Function5 ==
  send_to : TriggerPort  TriggerType=function-call  IsSimulinkFunction=on  FunctionName=send_to  FunctionVisibility=scoped  VariantControl=(inherit)
  u : ArgIn  DisableCoverage=on  ArgumentName=u
  Output : Outport
  wires:
  u/1 -> Output/1

== system VFlexP_small/Grid/Dynamic/Tertiary Control/MAS messages/ID7/Simulink Function6 ==
  Input1 : Inport
  Dest : TriggerPort  TriggerType=function-call  IsSimulinkFunction=on  FunctionName=Dest  FunctionVisibility=scoped  VariantControl=(inherit)
  Dest~ : ArgOut  DisableCoverage=on  ArgumentName=Dest
  wires:
  Input1/1 -> Dest~/1  "Dest"

== system VFlexP_small/Grid/Dynamic/Tertiary Control/MAS messages/ID7/Simulink Function7 ==
  set_following : TriggerPort  TriggerType=function-call  IsSimulinkFunction=on  FunctionName=set_following  FunctionVisibility=scoped  VariantControl=(inherit)
  u : ArgIn  DisableCoverage=on  ArgumentName=u
  Output : Outport
  wires:
  u/1 -> Output/1

== system VFlexP_small/Grid/Dynamic/Tertiary Control/MAS messages/ID7/Simulink Function8 ==
  type : TriggerPort  TriggerType=function-call  IsSimulinkFunction=on  FunctionName=type  FunctionVisibility=scoped  VariantControl=(inherit)
  Compare To Constant : simulink/Logic and Bit Operations/Compare To Constant  relop=~=  const=0  OutDataTypeStr=boolean  ZeroCross=off
  Send : Send  OutputPortMessageModes=m  ShowEnablePort=on
      settings: InputPortMap=e0,u1
  u : ArgIn  DisableCoverage=on  ArgumentName=u
  type_out : Outport
  trigger : Outport  Port=2
  wires:
  Send/1 -> trigger/1
  Compare To Constant/1 -> Send/2, Send/1
  u/1 -> type_out/1, Compare To Constant/1

== system VFlexP_small/Grid/Dynamic/Tertiary Control/MAS messages/ID7/Simulink Function9 ==
  Input1 : Inport
  get_leader : TriggerPort  TriggerType=function-call  IsSimulinkFunction=on  FunctionName=get_leader  FunctionVisibility=scoped  VariantControl=(inherit)
  value : ArgOut  ArgumentName=value
  wires:
  Input1/1 -> value/1

== system VFlexP_small/Grid/Dynamic/Tertiary Control/MAS messages/ID7/Subsystem ==
  In1 : Inport
  In3 : Inport  Port=2
  In4 : Inport  Port=3
  AND11 : Logic  IconShape=distinctive  AllPortsSameDT=off  OutDataTypeStr=boolean
  AND9 : Logic  IconShape=distinctive  AllPortsSameDT=off  OutDataTypeStr=boolean
  Compare To Zero : simulink/Logic and Bit Operations/Compare To Zero  relop=>  OutDataTypeStr=boolean
  Compare To Zero1 : simulink/Logic and Bit Operations/Compare To Zero  relop=<  OutDataTypeStr=boolean
  NOT : Logic  Operator=NOT  IconShape=distinctive  AllPortsSameDT=off  OutDataTypeStr=boolean
  OR4 : Logic  Operator=OR  IconShape=distinctive  AllPortsSameDT=off  OutDataTypeStr=boolean
  Relational Operator2 : RelationalOperator  Operator=<  OutDataTypeStr=boolean  RndMeth=Simplest  InputSameDT=off
  Relational Operator3 : RelationalOperator  Operator=>  OutDataTypeStr=boolean  RndMeth=Simplest  InputSameDT=off
  Out1 : Outport
  inf_satur : Outport  Port=2
  wires:
  In1/1 -> Compare To Zero/1, Compare To Zero1/1
  OR4/1 -> NOT/1
  Relational Operator2/1 -> AND9/1
  AND9/1 -> OR4/1
  In4/1 -> Relational Operator2/1, Relational Operator3/1
  AND11/1 -> inf_satur/1, OR4/2
  Relational Operator3/1 -> AND11/1
  In3/1 -> Relational Operator2/2, Relational Operator3/2
  Compare To Zero1/1 -> AND11/2
  Compare To Zero/1 -> AND9/2
  NOT/1 -> Out1/1

== system VFlexP_small/Grid/Dynamic/Tertiary Control/MAS messages/ID7/Triggered Subsystem ==
  In1 : Inport
  Trigger : TriggerPort  VariantControl=(inherit)
  Out1 : Outport
  wires:
  In1/1 -> Out1/1

== system VFlexP_small/Grid/Dynamic/Tertiary Control/MAS messages/ID7/Triggered Subsystem1 ==
  In1 : Inport
  Trigger : TriggerPort  VariantControl=(inherit)
  Out1 : Outport
  wires:
  In1/1 -> Out1/1

== system VFlexP_small/Grid/Dynamic/Tertiary Control/MAS messages/ID7/Triggered Subsystem2 ==
  In1 : Inport
  Trigger : TriggerPort  VariantControl=(inherit)
  Out1 : Outport
  wires:
  In1/1 -> Out1/1

== system VFlexP_small/Grid/Dynamic/Tertiary Control/MAS messages/ID7/Triggered Subsystem3 ==
  Trigger : TriggerPort  VariantControl=(inherit)
  One : Constant  OutDataTypeStr=Inherit: Inherit via back propagation
  Send7 : Send  OutputPortMessageModes=m  ShowEnablePort=on
      settings: InputPortMap=e0,u1
  Out1 : Outport
  wires:
  Send7/1 -> Out1/1
  One/1 -> Send7/2, Send7/1

== system VFlexP_small/Grid/Dynamic/Tertiary Control/MAS messages/ID7/Triggered Subsystem4 ==
  In1 : Inport
  Trigger : TriggerPort  VariantControl=(inherit)
  Out1 : Outport
  wires:
  In1/1 -> Out1/1

== system VFlexP_small/Grid/Dynamic/Tertiary Control/MAS messages/ID7/Triggered Subsystem5 ==
  In1 : Inport
  Trigger : TriggerPort  TriggerType=falling  VariantControl=(inherit)
  Constant : Constant
  IC : InitialCondition  Value=0
  Out1 : Outport
  Output : Outport  Port=2
  wires:
  In1/1 -> Out1/1
  Constant/1 -> IC/1
  IC/1 -> Output/1

== system VFlexP_small/Grid/Dynamic/Tertiary Control/MAS messages/ID7/Triggered Subsystem6 ==
  In1 : Inport
  Trigger : TriggerPort  VariantControl=(inherit)
  Out1 : Outport
  wires:
  In1/1 -> Out1/1

== system VFlexP_small/Grid/Dynamic/Tertiary Control/MAS messages/ID7/ramp ==
  connected : Inport
  time : Inport  Port=2
  Clock5 : Clock
      settings: DisableCoverage=on
  Gain : Gain  Gain=0.05
  Product : Product
  Sum6 : Sum  DisableCoverage=on  Inputs=|+-  InputSameDT=on  SaturateOnIntegerOverflow=on  OutDataTypeStr=Inherit: Same as first input
  Out1 : Outport
  wires:
  connected/1 -> Product/1
  Product/1 -> Gain/1
  Gain/1 -> Out1/1
  Sum6/1 -> Product/2
  time/1 -> Sum6/2
  Clock5/1 -> Sum6/1

== system VFlexP_small/Grid/Dynamic/Tertiary Control/MAS messages/ID7/time ==
  time : Inport
  Trigger : TriggerPort  VariantControl=(inherit)
  Out1 : Outport
  wires:
  time/1 -> Out1/1

== system VFlexP_small/Grid/Loadflow/Grid/Dynamic/Buses/dynamic ==
  i_d_in : Inport
  i_q_in : Inport  Port=2
  i_d_out : Inport  Port=3
  i_q_out : Inport  Port=4
  Gain1 : Gain  Gain=1./Rcf(bus_complexity_PF == 1)
  Gain2 : Gain  Gain=1./Rcf(bus_complexity_PF == 1)
  Gain3 : Gain  Gain=Cbuses(bus_complexity_PF == 1)
  Gain4 : Gain  Gain=Cbuses(bus_complexity_PF== 1)
  Gain5 : Gain  Gain=omegab./Cbuses(bus_complexity_PF == 1)
  Gain6 : Gain  Gain=omegab./Cbuses(bus_complexity_PF == 1)
  Product : Product
  Product1 : Product
  Selector{,1..3} (4 alike) : Selector  InputPortWidth=Nbuses  IndexOptions=Index vector (dialog)  Indices=find(bus_complexity_PF == 1)  OutputSizes=1
  Sum10 : Sum  Inputs=|-++
  Sum11 : Sum  Inputs=-+|
  Sum12 : Sum  Inputs=|+-
  Sum13 : Sum  Inputs=-+-|
  to_all_Nodes : Subsystem
  to_all_Nodes1 : Subsystem
  vd : Integrator  InitialCondition=1
  vq : Integrator
  v_d : Outport
  v_q : Outport  Port=2
  wires:
  Sum10/1 -> Gain6/1
  Gain3/1 -> Product1/1
  vq/1 -> to_all_Nodes1/1(In1), Gain2/1, Gain3/1  "vq"
  Product1/1 -> Sum10/3
  Gain4/1 -> Product/1
  Gain2/1 -> Sum13/3
  Product/1 -> Sum13/1
  Sum11/1 -> Sum10/2
  Gain6/1 -> vd/1
  [omega_ref] -> Product1/2, Product/2  "omega"
  Sum13/1 -> Gain5/1
  Gain1/1 -> Sum10/1
  Gain5/1 -> vq/1
  Sum12/1 -> Sum13/2
  vd/1 -> Gain4/1, to_all_Nodes/1(In1), Gain1/1  "vd"
  Selector/1 -> Sum11/2  "id1"
  Selector2/1 -> Sum11/1  "id2"
  Selector1/1 -> Sum12/1  "iq1"
  Selector3/1 -> Sum12/2  "iq2"
  i_d_in/1 -> Selector/1
  to_all_Nodes/1(Out1) -> v_d/1
  i_q_in/1 -> Selector1/1
  i_d_out/1 -> Selector2/1
  i_q_out/1 -> Selector3/1
  to_all_Nodes1/1(Out1) -> v_q/1

== system VFlexP_small/Grid/Loadflow/Grid/Dynamic/Buses/only R ==
  i_d_in : Inport
  i_q_in : Inport  Port=2
  i_d_out : Inport  Port=3
  i_q_out : Inport  Port=4
  Gain : Gain  Gain=Rcf(bus_complexity_PF == 4)
  Gain2 : Gain  Gain=Rcf(bus_complexity_PF == 4)
  Selector{,1..3} (4 alike) : Selector  InputPortWidth=Nbuses  IndexOptions=Index vector (dialog)  Indices=find(bus_complexity_PF == 4)  OutputSizes=1
  Sum1 : Sum  Inputs=|+-
  Sum2 : Sum  Inputs=|+-
  to_all_Nodes : Subsystem
  to_all_Nodes1 : Subsystem
  v_d : Outport
  v_q : Outport  Port=2
  wires:
  Selector1/1 -> Sum2/1  "iq1"
  Sum1/1 -> Gain/1  "id"
  Sum2/1 -> Gain2/1  "iq"
  Selector3/1 -> Sum2/2  "iq2"
  Selector/1 -> Sum1/1  "id"
  Selector2/1 -> Sum1/2
  Gain2/1 -> to_all_Nodes1/1(In1)
  Gain/1 -> to_all_Nodes/1(In1)
  to_all_Nodes/1(v_d) -> v_d/1
  to_all_Nodes1/1(v_d) -> v_q/1
  i_q_in/1 -> Selector1/1
  i_q_out/1 -> Selector3/1
  i_d_out/1 -> Selector2/1
  i_d_in/1 -> Selector/1

== system VFlexP_small/Grid/Loadflow/Grid/Dynamic/Buses/static ==
  i_d_in : Inport
  i_q_in : Inport  Port=2
  i_d_out : Inport  Port=3
  i_q_out : Inport  Port=4
  Constant : Constant  Value=(1./Rcf(bus_complexity_PF == 2)).^2  VectorParams1D=off
  Constant1 : Constant
  Divide : Product  Inputs=*/
  Gain : Gain  Gain=Cbuses(bus_complexity_PF == 2)
  Gain1 : Gain  Gain=1./Rcf(bus_complexity_PF == 2)
  Gain2 : Gain  Gain=1./Rcf(bus_complexity_PF == 2)
  Product{,1..5} (6 alike) : Product
  Selector{,1..3} (4 alike) : Selector  InputPortWidth=Nbuses  IndexOptions=Index vector (dialog)  Indices=find(bus_complexity_PF == 2)  OutputSizes=1
  Sum : Sum  Inputs=|++
  Sum1 : Sum  Inputs=|-+
  Sum2 : Sum  Inputs=|+-
  Sum3 : Sum  Inputs=|++
  Sum4 : Sum  Inputs=|-+
  to_all_Nodes : Subsystem
  to_all_Nodes1 : Subsystem
  v_d : Outport
  v_q : Outport  Port=2
  wires:
  Product5/1 -> Sum4/2
  Gain2/1 -> Product5/2
  Product4/1 -> Sum4/1
  Product2/1 -> Product3/1, Product4/2
  Product3/1 -> Sum3/2
  Product1/1 -> Sum3/1
  Divide/1 -> Product2/1, Gain1/1, Product5/1
  Gain1/1 -> Product1/2
  Sum2/1 -> Product3/2, Gain2/1  "iq"
  Sum1/1 -> Product4/1, Product1/1  "id"
  Constant1/1 -> Divide/1
  Product/1 -> Sum/2
  Gain/1 -> Product/1, Product/2, Product2/2
  Sum/1 -> Divide/2
  Constant/1 -> Sum/1
  Sum4/1 -> to_all_Nodes1/1(In1)  "vq"
  Sum3/1 -> to_all_Nodes/1(In1)  "vd"
  [omega_ref] -> Gain/1  "omega"
  Selector/1 -> Sum1/2  "id1"
  Selector2/1 -> Sum1/1  "id2"
  Selector1/1 -> Sum2/1  "iq1"
  Selector3/1 -> Sum2/2  "iq2"
  to_all_Nodes/1(v_d) -> v_d/1
  i_d_in/1 -> Selector/1
  i_q_in/1 -> Selector1/1
  i_q_out/1 -> Selector3/1
  to_all_Nodes1/1(v_q) -> v_q/1
  i_d_out/1 -> Selector2/1

== system VFlexP_small/Grid/Loadflow/Grid/Dynamic/Buses/static omega ==
  i_d_in : Inport
  i_q_in : Inport  Port=2
  i_d_out : Inport  Port=3
  i_q_out : Inport  Port=4
  Gain : Gain  Gain=1./((1./Rcf(bus_complexity_PF == 3)).^2+Cbuses(bus_complexity_PF == 3).^2)
  Gain1 : Gain  Gain=1./((1./Rcf(bus_complexity_PF == 3)).^2+Cbuses(bus_complexity_PF == 3).^2)
  Gain3 : Gain  Gain=1./Rcf(bus_complexity_PF == 3)
  Gain4 : Gain  Gain=Cbuses(bus_complexity_PF == 3)
  Gain5 : Gain  Gain=1./Rcf(bus_complexity_PF == 3)
  Gain6 : Gain  Gain=Cbuses(bus_complexity_PF == 3)
  Selector{,1..3} (4 alike) : Selector  InputPortWidth=Nbuses  IndexOptions=Index vector (dialog)  Indices=find(bus_complexity_PF == 3)  OutputSizes=1
  Sum : Sum  Inputs=|++
  Sum1 : Sum  Inputs=|+-
  Sum2 : Sum  Inputs=|+-
  Sum4 : Sum  Inputs=|-+
  to_all_Nodes : Subsystem
  to_all_Nodes1 : Subsystem
  v_d : Outport
  v_q : Outport  Port=2
  wires:
  Selector1/1 -> Sum2/1  "iq1"
  Sum1/1 -> Gain/1  "id"
  Sum2/1 -> Gain1/1  "iq"
  Selector3/1 -> Sum2/2  "iq2"
  Selector/1 -> Sum1/1  "id"
  Selector2/1 -> Sum1/2
  Gain/1 -> Gain3/1, Gain4/1
  Gain1/1 -> Gain5/1, Gain6/1
  Gain3/1 -> Sum/1
  Gain6/1 -> Sum/2
  Gain4/1 -> Sum4/1
  Gain5/1 -> Sum4/2
  Sum4/1 -> to_all_Nodes1/1(In1)
  Sum/1 -> to_all_Nodes/1(In1)
  i_q_out/1 -> Selector3/1
  i_q_in/1 -> Selector1/1
  to_all_Nodes/1(v_d) -> v_d/1
  i_d_in/1 -> Selector/1
  i_d_out/1 -> Selector2/1
  to_all_Nodes1/1(v_q) -> v_q/1
